simulink model "ExampleAddPhysics"  (Simulink 9.2)
settings: Solver=FixedStepDiscrete  StartTime=0.0  StopTime=10.0  FixedStep=" 0.0025"  RelTol=1e-3  EnableMultiTasking=on
libraries: rFproPhysicsLib x3
Description:
  | Compiled Plugin Only
settings Model: Creator=enewton  LastModifiedBy=SeanKavanagh
settings OptimizationCC: ExpressionDepthLimit=2147483647  AccelVerboseBuild=on
settings DebuggingCC: SolverPrmCheckMsg=warning  InheritedTsInSrcMsg=none
settings HardwareCC: TargetBitPerPointer=64  TargetBitPerSizeT=64  TargetBitPerPtrDiffT=64  TargetLongLongMode=on  TargetIntDivRoundTo=Zero  TargetEndianess=LittleEndian  TargetWordSize=64  TargetHWDeviceType=MATLAB Host  ProdEqTarget=off
settings RTWCC: SystemTargetFile=rfpro.tlc  MakeCommand="make_rtw OPTS=\"-DADD_PHYSICS\""  TemplateMakefile=rfpro.tmf  Description=rFpro Target (Add Physics)  TargetLang=C++
settings STFCustomTargetCC: ModelReferenceCompliant=off  GeneratePreprocessorConditionals=Disable all  CombineOutputUpdateFcns=on  MatFileLogging=on  CPPClassGenCompliant=on  GRTInterface=off  SystemTargetFile=rfpro.tlc
settings GRTTargetCC: ModelReferenceCompliant=off  ParMdlRefBuildCompliant=off  CompOptLevelCompliant=off  ConcurrentExecutionCompliant=off  CombineOutputUpdateFcns=on  GRTInterface=off  UseToolchainInfoCompliant=off

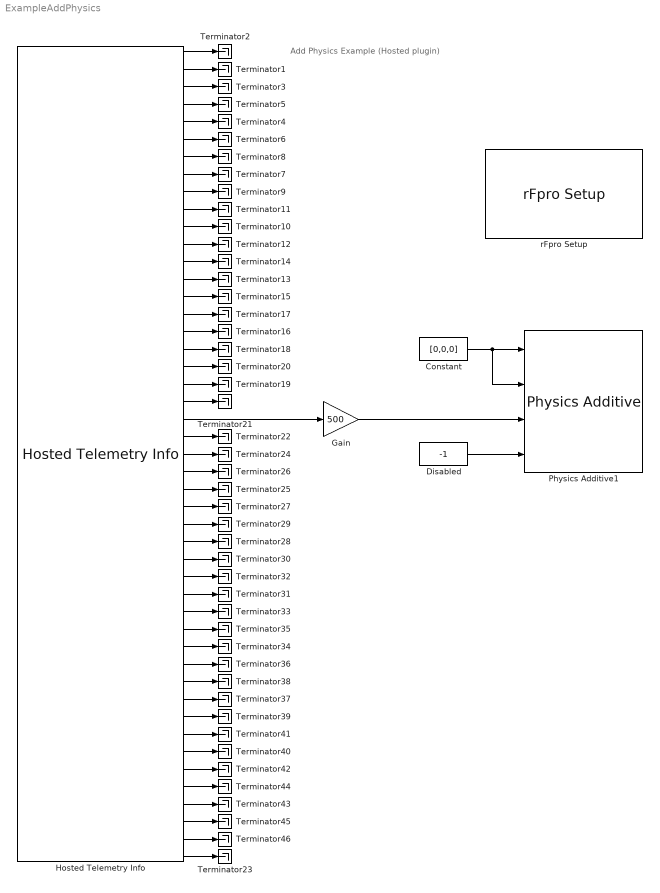
== system ExampleAddPhysics ==
  note: Add Physics Example (Hosted plugin)
  Constant : Constant  Value=[0,0,0]
  Disabled : Constant  Value=-1
  Gain : Gain  Gain=500
  Hosted Telemetry Info : rFproPhysicsLib/Hosted Blocks/Hosted Telemetry Info  SFunctionModules=''
  Physics Additive1 : rFproPhysicsLib/Hosted Blocks/Physics Additive
  Terminator{1..46} (46 alike) : Terminator
  rFpro Setup : rFproPhysicsLib/rFpro Setup  Priority=1  platform=Hosted Plugin  stopOnSessionEnd=on  usePseudoRealtime=on  syncToRF=on  useReverseByteOrder=off  useRfTime=on  minIterations=4  maxIterations=1000  ipReceiveAddress='127.0.0.1'  ipReceivePort=11054  receiveSampleTime=-1  ipTransmitAddress='127.0.0.1'  ipTransmitPort=11052  transmitSampleTime=-1  pluginType=ADD_PHYSICS
  wires:
  Hosted Telemetry Info/22 -> Gain/1
  Gain/1 -> Physics Additive1/3
  Disabled/1 -> Physics Additive1/4
  Hosted Telemetry Info/1 -> Terminator2/1
  Hosted Telemetry Info/2 -> Terminator1/1
  Hosted Telemetry Info/3 -> Terminator3/1
  Hosted Telemetry Info/4 -> Terminator5/1
  Hosted Telemetry Info/5 -> Terminator4/1
  Hosted Telemetry Info/6 -> Terminator6/1
  Hosted Telemetry Info/7 -> Terminator8/1
  Hosted Telemetry Info/8 -> Terminator7/1
  Hosted Telemetry Info/9 -> Terminator9/1
  Hosted Telemetry Info/10 -> Terminator11/1
  Hosted Telemetry Info/11 -> Terminator10/1
  Hosted Telemetry Info/12 -> Terminator12/1
  Hosted Telemetry Info/13 -> Terminator14/1
  Hosted Telemetry Info/14 -> Terminator13/1
  Hosted Telemetry Info/15 -> Terminator15/1
  Hosted Telemetry Info/16 -> Terminator17/1
  Hosted Telemetry Info/17 -> Terminator16/1
  Hosted Telemetry Info/18 -> Terminator18/1
  Hosted Telemetry Info/19 -> Terminator20/1
  Hosted Telemetry Info/20 -> Terminator19/1
  Hosted Telemetry Info/21 -> Terminator21/1
  Hosted Telemetry Info/23 -> Terminator22/1
  Hosted Telemetry Info/24 -> Terminator24/1
  Hosted Telemetry Info/25 -> Terminator26/1
  Hosted Telemetry Info/26 -> Terminator25/1
  Hosted Telemetry Info/27 -> Terminator27/1
  Hosted Telemetry Info/28 -> Terminator29/1
  Hosted Telemetry Info/29 -> Terminator28/1
  Hosted Telemetry Info/30 -> Terminator30/1
  Hosted Telemetry Info/31 -> Terminator32/1
  Hosted Telemetry Info/32 -> Terminator31/1
  Hosted Telemetry Info/33 -> Terminator33/1
  Hosted Telemetry Info/34 -> Terminator35/1
  Hosted Telemetry Info/35 -> Terminator34/1
  Hosted Telemetry Info/36 -> Terminator36/1
  Hosted Telemetry Info/37 -> Terminator38/1
  Hosted Telemetry Info/38 -> Terminator37/1
  Hosted Telemetry Info/39 -> Terminator39/1
  Hosted Telemetry Info/40 -> Terminator41/1
  Hosted Telemetry Info/41 -> Terminator40/1
  Hosted Telemetry Info/42 -> Terminator42/1
  Hosted Telemetry Info/43 -> Terminator44/1
  Hosted Telemetry Info/44 -> Terminator43/1
  Hosted Telemetry Info/45 -> Terminator45/1
  Hosted Telemetry Info/46 -> Terminator46/1
  Constant/1 -> Physics Additive1/2, Physics Additive1/1
  Hosted Telemetry Info/47 -> Terminator23/1
